simulink subsystem "Cntct"  (R2021b)
settings: Solver=VariableStepAuto  StartTime=0.0  StopTime=10.0  RelTol=1e-3
settings Model: Creator=whamada  LastModifiedBy=whamada

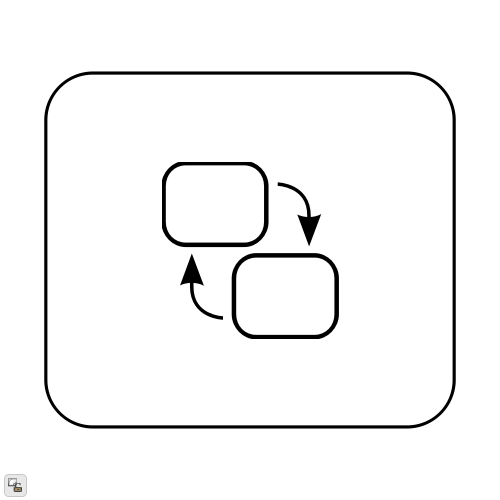
[thumbnail: Simulink's stored preview of the top-level diagram]
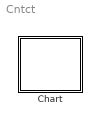
== system Cntct ==
  Chart : Stateflow chart  TreatAsAtomicUnit=on

== stateflow chart Cntct/Chart ==
